simulink model "muscle_twitch"  (R2021a)
settings: Solver=VariableStepAuto  StartTime=0.0  StopTime=5  RelTol=1e-3
settings Model: Creator=PUGAZH  LastModifiedBy=PUGAZH

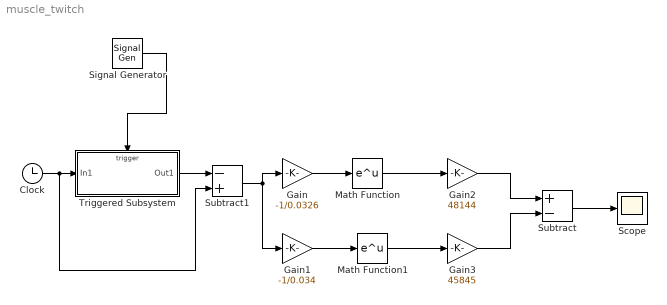
== system muscle_twitch ==
  Clock : Clock
  Gain : Gain  Gain=-1/0.0326
  Gain1 : Gain  Gain=-1/0.034
  Gain2 : Gain  Gain=48144
  Gain3 : Gain  Gain=45845
  Math Function : Math  SaturateOnIntegerOverflow=on
  Math Function1 : Math  SaturateOnIntegerOverflow=on
  Scope : Scope
  Signal Generator : SignalGenerator  Frequency=5
  Subtract : Sum  Inputs=+-
  Subtract1 : Sum  Inputs=-+
  Triggered Subsystem : Subsystem  TreatAsAtomicUnit=on
  wires:
  Gain/1 -> Math Function/1
  Gain1/1 -> Math Function1/1
  Math Function/1 -> Gain2/1
  Math Function1/1 -> Gain3/1
  Gain2/1 -> Subtract/1
  Gain3/1 -> Subtract/2
  Subtract/1 -> Scope/1
  Signal Generator/1 -> Triggered Subsystem/Trigger
  Subtract1/1 -> Gain1/1, Gain/1
  Triggered Subsystem/1(Out1) -> Subtract1/1
  Clock/1 -> Subtract1/2, Triggered Subsystem/1(In1)

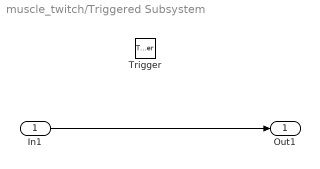
== system muscle_twitch/Triggered Subsystem ==
  In1 : Inport
  Trigger : TriggerPort  VariantControl=(inherit)
  Out1 : Outport
  wires:
  In1/1 -> Out1/1
